simulink model "Book4132"  (R2019b)
settings: Solver=ode4  StartTime=0  StopTime=10.0  FixedStep=0.001  RelTol=1e-3  EnableMultiTasking=on
settings Model: Creator=xyh  LastModifiedBy=user
settings DataIOCC: ReturnWorkspaceOutputs=off
settings OptimizationCC: LifeSpan=inf
settings DebuggingCC: SFUnexpectedBacktrackingDiag=warning  SFNoUnconditionalDefaultTransitionDiag=warning  ArithmeticOperatorsInVariantConditions=warning
settings SFSimCC: SimUseLocalCustomCode=off  CustomCodeUndefinedFunction=UseInterfaceOnly
settings RTWCC: RTWUseLocalCustomCode=off
settings CodeAppCC: StateflowObjectComments=on
settings GRTTargetCC: TargetLangStandard=C89/C90 (ANSI)  GeneratePreprocessorConditionals=Disable all
settings ConfigComp: CovMetricSettings=dw  CovHtmlReporting=on  CovSaveCumulativeToWorkspaceVar=on  CovSaveSingleToWorkspaceVar=on  CovExternalEMLEnable=off

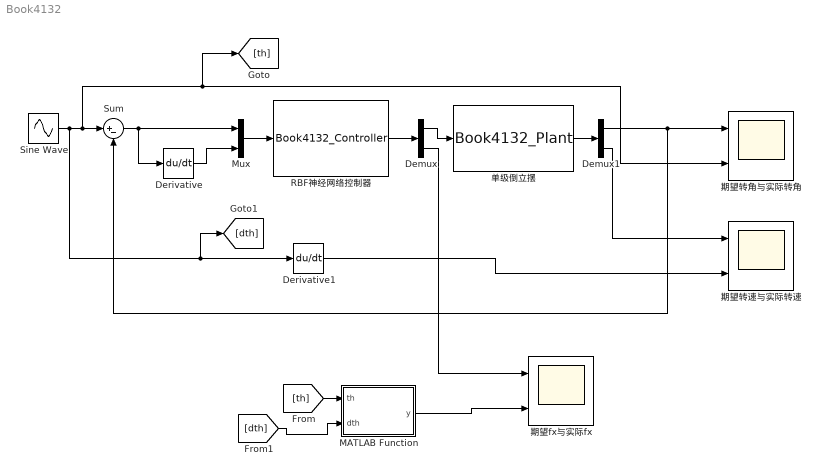
== system Book4132 ==
  Demux : Demux  Outputs=2
  Demux1 : Demux  Outputs=2
  Derivative : Derivative
  Derivative1 : Derivative
  MATLAB Function : MATLAB Function  TreatAsAtomicUnit=on
  Mux : Mux  Inputs=2
  RBF神经网络控制器 : S-Function  FunctionName=Book4132_Controller  SFunctionDeploymentMode=off  EnableBusSupport=off
  Sine Wave : Sin  Amplitude=0.1  SampleTime=0
  Sum : Sum  Inputs=|+-
  单级倒立摆 : S-Function  FunctionName=Book4132_Plant  SFunctionDeploymentMode=off  EnableBusSupport=off
  期望fx与实际fx : Scope  NumInputPorts=2
  期望转角与实际转角 : Scope  NumInputPorts=2
  期望转速与实际转速 : Scope  NumInputPorts=2
  wires:
  Mux/1 -> RBF神经网络控制器/1
  Demux1/1 -> 期望转角与实际转角/1, Sum/2
  Sine Wave/1 -> [dth], Derivative1/1, [th], 期望转角与实际转角/2, Sum/1
  Sum/1 -> Derivative/1, Mux/1
  Derivative/1 -> Mux/2
  RBF神经网络控制器/1 -> Demux/1
  Demux/1 -> 单级倒立摆/1
  单级倒立摆/1 -> Demux1/1
  Demux1/2 -> 期望转速与实际转速/1
  Derivative1/1 -> 期望转速与实际转速/2
  Demux/2 -> 期望fx与实际fx/1
  [th] -> MATLAB Function/1(th)
  [dth] -> MATLAB Function/2(dth)
  MATLAB Function/1(y) -> 期望fx与实际fx/2

== matlab function Book4132/MATLAB Function ==
  data: th input; y output; dth input
function y = fcn(th, dth)
%#codegen
g = 9.8;
mc = 1;     %小车质量
m = 0.1;    %摆的质量
l = 0.5;
f_up = g*sin(th) - m*l*dth^2*cos(th)*sin(th)/(mc+m);
f_down = l *(4/3 - m*(cos(th)^2)/(mc+m));
f = f_up / f_down;
y = f;
